simulink model "Servo_Simulink"  (R2022b)
settings: Solver=FixedStepDiscrete  StartTime=0.0  StopTime=50.0  FixedStep=0.1  RelTol=1e-3
libraries: jMPClib x2
settings Model: Creator=Jonathan Currie  LastModifiedBy=Jonathan Currie

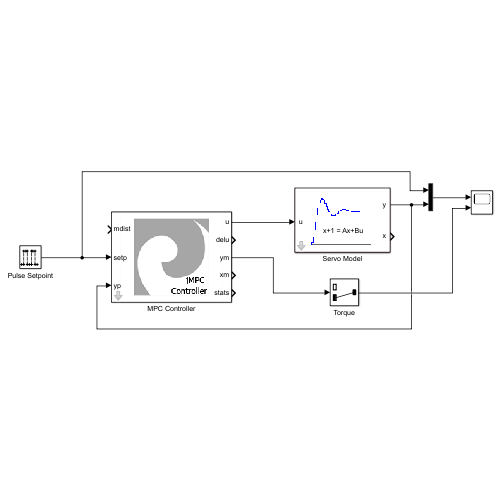
[thumbnail: Simulink's stored preview of the top-level diagram]
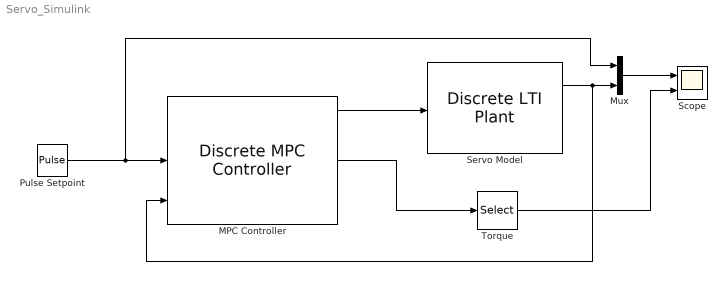
== system Servo_Simulink ==
  MPC Controller : jMPClib/MPC Blocks/Discrete MPC Controller  SIMJMPC=MPC1
      settings: SourceProductName=JMPC Toolbox
  Mux : Mux  Inputs=2
  Pulse Setpoint : DiscretePulseGenerator  Period=400  PulseWidth=200  SampleTime=0.1
  Scope : Scope  NumInputPorts=2
  Servo Model : jMPClib/MPC Blocks/Discrete LTI Plant  jSSobj=Plant
      settings: SourceProductName=JMPC Toolbox
  Torque : Selector  InputPortWidth=2  IndexOptions=Index vector (dialog)  Indices=2  OutputSizes=1
  wires:
  MPC Controller/1 -> Servo Model/1
  Servo Model/1 -> MPC Controller/3, Mux/2
  Pulse Setpoint/1 -> Mux/1, MPC Controller/2
  MPC Controller/3 -> Torque/1
  Mux/1 -> Scope/1
  Torque/1 -> Scope/2
